simulink model "Dynamic_Model_Simulink"  (R2022a)
settings: Solver=VariableStepAuto  StartTime=0.0  StopTime=1200  MaxStep=0.001  RelTol=1e-3
values from neighbouring files (symbols this model uses):
  B_F = 10000    [Dynamic_Model.m]
  Battery_Voltage = 364    [Dynamic_Model.m]
  Cd = 0.28    [Dynamic_Model.m]
  Crr = 0.015    [Dynamic_Model.m]
  GR = 7.8    [Dynamic_Model.m]
  GVM = (Vm+Dm)    (= 1790)    [Dynamic_Model.m]
  GVW = (Vm+Dm)*g    (= 17559.9)    [Dynamic_Model.m]
  M_Eff = Motor(2:16,2:16)    [Dynamic_Model.m]
  M_Regen_Eff = Motor_Regen(2:16,2:16)    [Dynamic_Model.m]
  M_Regen_Speed = Motor_Regen(2:16,1)    [Dynamic_Model.m]
  M_Regen_Torque = Motor_Regen(2:16,17)    [Dynamic_Model.m]
  M_Speed = Motor(2:16,1)    [Dynamic_Model.m]
  M_Torque = Motor(2:16,17)    [Dynamic_Model.m]
  MC_Eff = Motor_C(2:16,2:16)    [Dynamic_Model.m]
  MC_Regen_Eff = Motor_C_Regen(2:16,2:16)    [Dynamic_Model.m]
  MC_Regen_Speed = Motor_C_Regen(2:16,1)    [Dynamic_Model.m]
  MC_Regen_Torque = Motor_C_Regen(2:16,17)    [Dynamic_Model.m]
  MC_Speed = Motor_C(2:16,1)    [Dynamic_Model.m]
  MC_Torque = Motor_C(2:16,17)    [Dynamic_Model.m]
  P_Avl = 30000    [Dynamic_Model.m]
  Rho = 1.225    [Dynamic_Model.m]
  Rw = 0.2032    [Dynamic_Model.m]
  theta = 0    [Dynamic_Model.m]
  Va = 3.8056    [Dynamic_Model.m]
libraries: slpidlib x1
settings Model: Creator=sujee  LastModifiedBy=sujee

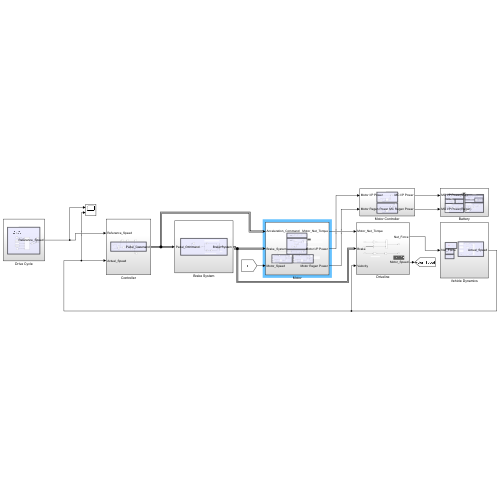
[thumbnail: Simulink's stored preview of the top-level diagram]
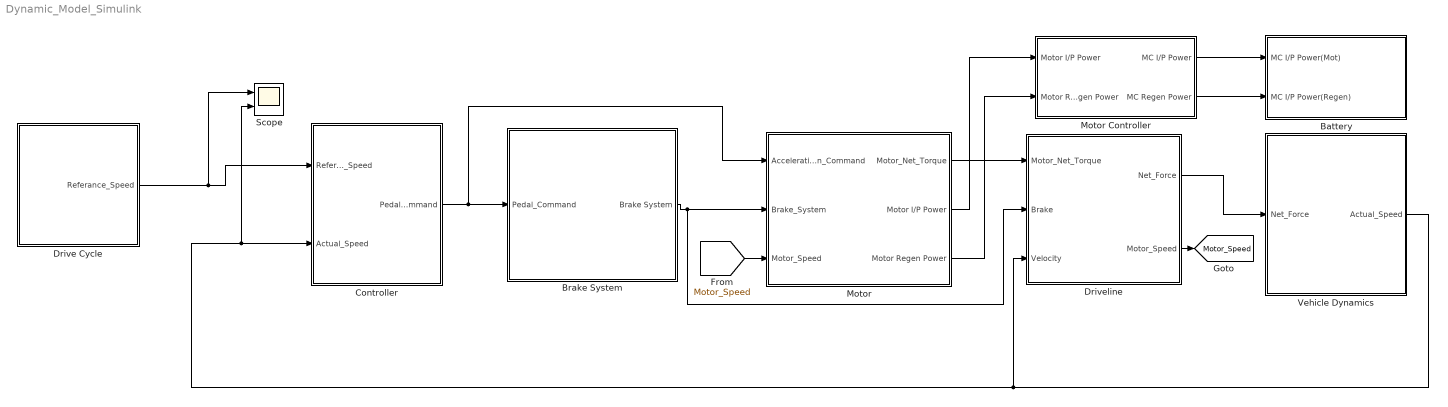
== system Dynamic_Model_Simulink ==
  Battery : Subsystem
  Brake System : Subsystem
  Controller : Subsystem
  Drive Cycle : Subsystem
  Driveline : Subsystem
  Motor : Subsystem
  Motor Controller : Subsystem
  Scope : Scope  NumInputPorts=2
  Vehicle Dynamics : Subsystem
  tag scope: Motor_Speed=global
  wires:
  Vehicle Dynamics/1(Actual_Speed) -> Scope/2, Controller/2(Actual_Speed), Driveline/3(Velocity)
  Drive Cycle/1(Referance_Speed) -> Scope/1, Controller/1(Referance_Speed)
  Controller/1(Pedal_Command) -> Motor/1(Acceleration_Command), Brake System/1(Pedal_Command)
  Brake System/1(Brake System) -> Driveline/2(Brake), Motor/2(Brake_System)
  Motor/1(Motor_Net_Torque) -> Driveline/1(Motor_Net_Torque)
  Driveline/1(Net_Force) -> Vehicle Dynamics/1(Net_Force)
  Driveline/2(Motor_Speed) -> [Motor_Speed]
  [Motor_Speed] -> Motor/3(Motor_Speed)
  Motor/2(Motor I/P Power) -> Motor Controller/1(Motor I/P Power)
  Motor/3(Motor Regen Power) -> Motor Controller/2(Motor Regen Power)
  Motor Controller/1(MC I/P Power) -> Battery/1(MC I/P Power(Mot))
  Motor Controller/2(MC Regen Power) -> Battery/2(MC I/P Power(Regen))

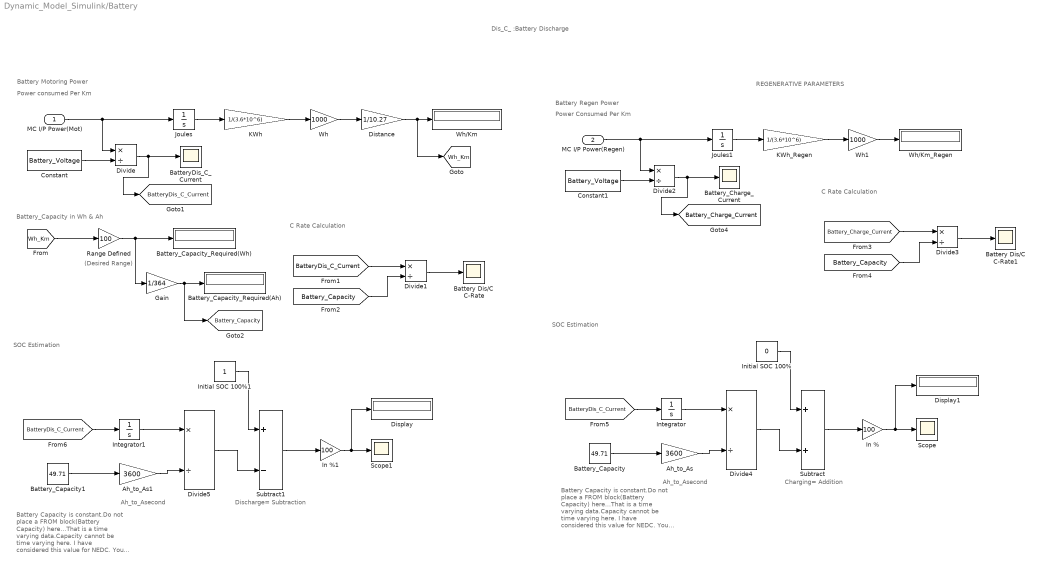
== system Dynamic_Model_Simulink/Battery ==
  note: Charging= Addition
  note: REGENERATIVE PARAMETERS
  note: SOC Estimation
  note: (Desired Range)
  note: Battery Motoring Power
  note: Battery Regen Power
  note: Dis_C_ :Battery Discharge
  note: C Rate Calculation
  note: Battery_Capacity in Wh & Ah
  note: Power consumed Per Km
  note: Power Consumed Per Km
  note: C Rate Calculation
  note: Ah_to_Asecond
  note: Battery Capacity is constant.Do not place a FROM block(Battery Capacity) here...That is a time varying data.Capacity cannot be time varying here.
      | I have considered this value for NEDC. You might get a diff value for other drive cycles, dynamically change the value here!
  note: Battery Capacity is constant.Do not place a FROM block(Battery Capacity) here...That is a time varying data.Capacity cannot be time varying here.
      | I have considered this value for NEDC. You might get a diff value for other drive cycles, dynamically change the value here!
  note: SOC Estimation
  note: Discharge= Subtraction
  note: Ah_to_Asecond
  MC I/P Power(Mot) : Inport
  MC I/P Power(Regen) : Inport  Port=2
  Ah_to_As : Gain  Gain=3600
  Ah_to_As1 : Gain  Gain=3600
  Battery Dis/C C-Rate : Scope
  Battery Dis/C C-Rate1 : Scope
  BatteryDis_C_Current : Scope
  Battery_Capacity : Constant  Value=49.71
  Battery_Capacity1 : Constant  Value=49.71
  Battery_Capacity_Required(Ah) : Display
  Battery_Capacity_Required(Wh) : Display
  Battery_Charge_Current : Scope
  Constant : Constant  Value=Battery_Voltage  VectorParams1D=off
  Constant1 : Constant  Value=Battery_Voltage  VectorParams1D=off
  Display : Display
  Display1 : Display
  Distance : Gain  Gain=1/10.27
  Divide{,1..5} (6 alike) : Product  Inputs=*/
  Gain : Gain  Gain=1/364
  In % : Gain  Gain=100
  In %1 : Gain  Gain=100
  Initial SOC 100% : Constant  Value=0
  Initial SOC 100%1 : Constant
  Integrator : Integrator
  Integrator1 : Integrator
  Joules : Integrator
  Joules1 : Integrator
  KWh : Gain  Gain=1/(3.6*10^6)
  KWh_Regen : Gain  Gain=1/(3.6*10^6)
  Range Defined : Gain  Gain=100
  Scope : Scope
  Scope1 : Scope
  Subtract : Sum
  Subtract1 : Sum  Inputs=+-
  Wh : Gain  Gain=1000
  Wh/Km : Display
  Wh/Km_Regen : Display
  Wh1 : Gain  Gain=1000
  tag scope: BatteryDis_C_Current=global, Battery_Capacity=global, Battery_Charge_Current=global, Wh_Km=global
  wires:
  MC I/P Power(Mot)/1 -> Joules/1, Divide/1
  Constant/1 -> Divide/2
  Joules/1 -> KWh/1
  KWh/1 -> Wh/1
  Wh/1 -> Distance/1
  Distance/1 -> [Wh_Km], Wh/Km/1
  [Wh_Km] -> Range Defined/1
  Range Defined/1 -> Battery_Capacity_Required(Wh)/1, Gain/1
  Divide/1 -> [BatteryDis_C_Current], BatteryDis_C_Current/1
  Gain/1 -> [Battery_Capacity], Battery_Capacity_Required(Ah)/1
  [BatteryDis_C_Current] -> Divide1/1
  [Battery_Capacity] -> Divide1/2
  Divide1/1 -> Battery Dis/C C-Rate/1
  MC I/P Power(Regen)/1 -> Joules1/1, Divide2/1
  Joules1/1 -> KWh_Regen/1
  Constant1/1 -> Divide2/2
  Divide2/1 -> [Battery_Charge_Current], Battery_Charge_Current/1
  KWh_Regen/1 -> Wh1/1
  Wh1/1 -> Wh/Km_Regen/1
  [Battery_Charge_Current] -> Divide3/1
  Divide3/1 -> Battery Dis/C C-Rate1/1
  [Battery_Capacity] -> Divide3/2
  Integrator/1 -> Divide4/1
  Battery_Capacity/1 -> Ah_to_As/1
  Initial SOC 100%/1 -> Subtract/1
  Divide4/1 -> Subtract/2
  In %/1 -> Display1/1, Scope/1
  Subtract/1 -> In %/1
  Ah_to_As/1 -> Divide4/2
  [BatteryDis_C_Current] -> Integrator/1
  Battery_Capacity1/1 -> Ah_to_As1/1
  Divide5/1 -> Subtract1/2
  Subtract1/1 -> In %1/1
  Initial SOC 100%1/1 -> Subtract1/1
  Integrator1/1 -> Divide5/1
  Ah_to_As1/1 -> Divide5/2
  [BatteryDis_C_Current] -> Integrator1/1
  In %1/1 -> Display/1, Scope1/1

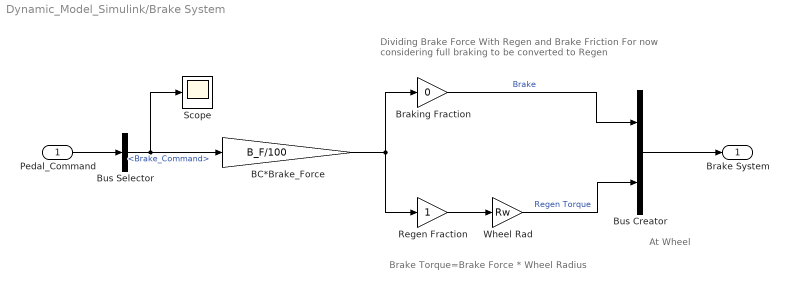
== system Dynamic_Model_Simulink/Brake System ==
  note: Dividing Brake Force With Regen and Brake Friction
      | For now considering full braking to be converted to Regen
  note: Brake Torque=Brake Force * Wheel Radius
  note: At Wheel
  Pedal_Command : Inport
  " Regen Fraction" : Gain
  BC*Brake_Force : Gain  Gain=B_F/100
  "Braking Fraction " : Gain  Gain=0
  Bus Creator : BusCreator  Inputs=2
  Bus Selector : BusSelector  OutputSignals=Brake_Command
  Scope : Scope
  Wheel Rad : Gain  Gain=Rw
  Brake System : Outport
  wires:
  Pedal_Command/1 -> Bus Selector/1
  Bus Selector/1 -> Scope/1, BC*Brake_Force/1  "<Brake_Command>"
  BC*Brake_Force/1 -> "Braking Fraction "/1, " Regen Fraction"/1
  " Regen Fraction"/1 -> Wheel Rad/1
  "Braking Fraction "/1 -> Bus Creator/1  "Brake"
  Wheel Rad/1 -> Bus Creator/2  "Regen Torque"
  Bus Creator/1 -> Brake System/1

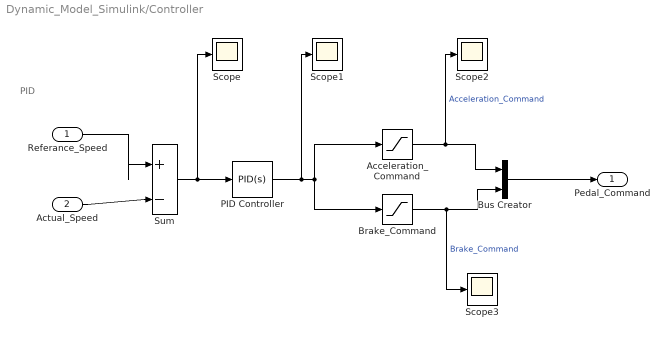
== system Dynamic_Model_Simulink/Controller ==
  note: PID
  Referance_Speed : Inport
  Actual_Speed : Inport  Port=2
  Acceleration_Command : Saturate  UpperLimit=inf  LowerLimit=0
  Brake_Command : Saturate  UpperLimit=0  LowerLimit=-inf
  Bus Creator : BusCreator  Inputs=2
  PID Controller : slpidlib/PID Controller  Controller=PID  Form=Parallel  TimeDomain=Continuous-time  UseExternalTs=off  SampleTime=-1  IntegratorMethod=Forward Euler  FilterMethod=Forward Euler  ControllerParametersSource=internal  P=200  I=1  UseKiTs=off  D=1  N=100  UseFilter=on  TunerSelectOption=Transfer Function Based (PID Tuner App)  InitialConditionSource=internal  InitialConditionForIntegrator=0  InitialConditionForFilter=0  DifferentiatorICPrevScaledInput=0  ExternalReset=none  TrackingMode=off  Kt=1  LimitOutput=off  SatLimitsSource=internal  UpperSaturationLimit=inf  LowerSaturationLimit=-inf  LinearizeAsGain=on  AntiWindupMode=none  Kb=1  POutMin=[]  POutMax=[]  IOutMin=[]  IOutMax=[]  DOutMin=[]  DOutMax=[]  NOutMin=[]  NOutMax=[]  SumOutMin=[]  SumOutMax=[]  SaturationOutMin=[]  SaturationOutMax=[]  PParamMin=[]  PParamMax=[]  IParamMin=[]  IParamMax=[]  DParamMin=[]  DParamMax=[]  NParamMin=[]  NParamMax=[]  KbParamMin=[]  KbParamMax=[]  KtParamMin=[]  KtParamMax=[]  KbOutMin=[]  KbOutMax=[]  KtOutMin=[]  KtOutMax=[]  IntegratorOutMin=[]  IntegratorOutMax=[]  FilterOutMin=[]  FilterOutMax=[]  SumI1OutMin=[]  SumI1OutMax=[]  SumI2OutMin=[]  SumI2OutMax=[]  SumI3OutMin=[]  SumI3OutMax=[]  SumI4OutMin=[]  SumI4OutMax=[]  SumDOutMin=[]  SumDOutMax=[]  DifferentiatorOutMin=[]  DifferentiatorOutMax=[]  FilterDiffOutCoefMin=[]  FilterDiffOutCoefMax=[]  ReciprocalOutMin=[]  ReciprocalOutMax=[]  SumDenOutMin=[]  SumDenOutMax=[]  SumNumOutMin=[]  SumNumOutMax=[]  DivideOutMin=[]  DivideOutMax=[]  UdiffTsProdOutMin=[]  UdiffTsProdOutMax=[]  NTsProdOutMin=[]  NTsProdOutMax=[]  UintegralTsProdOutMin=[]  UintegralTsProdOutMax=[]  UngainTsProdOutMin=[]  UngainTsProdOutMax=[]  IntegratorContinuousStateAttributes=''  IntegratorStateMustResolveToSignalObject=off  IntegratorRTWStateStorageClass=Auto  FilterContinuousStateAttributes=''  FilterStateMustResolveToSignalObject=off  FilterRTWStateStorageClass=Auto  ParallelPVariant=InternalParameters  IdealPVariant=Disabled  IVariant=InternalParameters  DVariant=InternalParameters  IntegratorVariant=Continuous  SatVariant=Disabled  AWVariant=Passthrough  PCopyVariant=Disabled  TRVariant=Disabled  FdbkBlocksVariant=Forward  IdealPFdbkVariant=Disabled  SatFdbkVariant=Disabled  DerivativeFilterVariant=ContFilter  NVariant=InternalParameters  NCopyVariant=Disabled  FilterICVariant=InternalICsFilter  IntegratorICVariant=InternalICs  ExternalResetVariant=Disabled  TRSumVariant=Passthrough  SumFdbkVariant=Disabled  SumVariant=Sum_PID  TsampFilterVariant=InternalTs  TsampNgainVariant=Passthrough  TsampIntegralVariant=Passthrough  ExternalSaturationOutDataTypeStr=Inherit: Same as second input  aMode=0
  Scope{,1..3} (4 alike) : Scope
  Sum : Sum  Inputs=|+-
  Pedal_Command : Outport
  wires:
  Referance_Speed/1 -> Sum/1
  Actual_Speed/1 -> Sum/2
  Sum/1 -> Scope/1, PID Controller/1
  PID Controller/1 -> Scope1/1, Brake_Command/1, Acceleration_Command/1
  Acceleration_Command/1 -> Scope2/1, Bus Creator/1  "Acceleration_Command"
  Brake_Command/1 -> Scope3/1, Bus Creator/2  "Brake_Command"
  Bus Creator/1 -> Pedal_Command/1

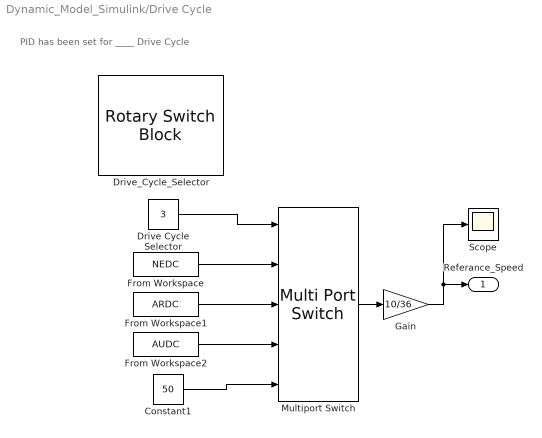
== system Dynamic_Model_Simulink/Drive Cycle ==
  note: PID has been set for ____ Drive Cycle
  Constant1 : Constant  Value=50
  Drive Cycle Selector : Constant  Value=3
  Drive_Cycle_Selector : RotarySwitchBlock
      settings: Values={{'NEDC', 'ARDC', 'AUDC', '60 m/s'}, [1 2 3 4]}
  From Workspace : FromWorkspace  VariableName=NEDC
  From Workspace1 : FromWorkspace  VariableName=ARDC
  From Workspace2 : FromWorkspace  VariableName=AUDC
  Gain : Gain  Gain=10/36
  Multiport Switch : MultiPortSwitch  Inputs=4  SaturateOnIntegerOverflow=off  InputSameDT=off
  Scope : Scope
  Referance_Speed : Outport
  wires:
  From Workspace/1 -> Multiport Switch/2
  From Workspace2/1 -> Multiport Switch/4
  From Workspace1/1 -> Multiport Switch/3
  Drive Cycle Selector/1 -> Multiport Switch/1
  Multiport Switch/1 -> Gain/1
  Constant1/1 -> Multiport Switch/5
  Gain/1 -> Scope/1, Referance_Speed/1

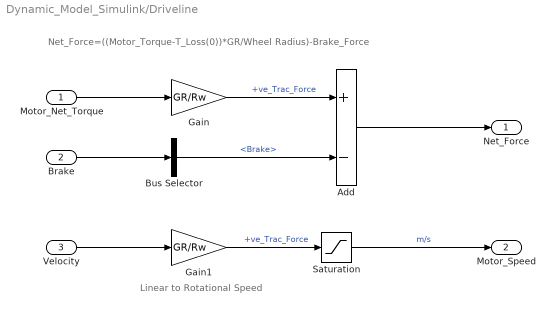
== system Dynamic_Model_Simulink/Driveline ==
  note: Linear to Rotational Speed
  note: Net_Force=((Motor_Torque-T_Loss(0))*GR/Wheel Radius)-Brake_Force
  Motor_Net_Torque : Inport
  Brake : Inport  Port=2
  Velocity : Inport  Port=3
  Add : Sum  Inputs=+-
  Bus Selector : BusSelector  OutputSignals=Brake
  Gain : Gain  Gain=GR/Rw
  Gain1 : Gain  Gain=GR/Rw
  Saturation : Saturate  UpperLimit=inf  LowerLimit=0.00001
  Net_Force : Outport
  Motor_Speed : Outport  Port=2
  wires:
  Motor_Net_Torque/1 -> Gain/1
  Gain/1 -> Add/1  "+ve_Trac_Force"
  Brake/1 -> Bus Selector/1
  Bus Selector/1 -> Add/2  "<Brake>"
  Velocity/1 -> Gain1/1
  Gain1/1 -> Saturation/1  "+ve_Trac_Force"
  Add/1 -> Net_Force/1
  Saturation/1 -> Motor_Speed/1  "m/s"

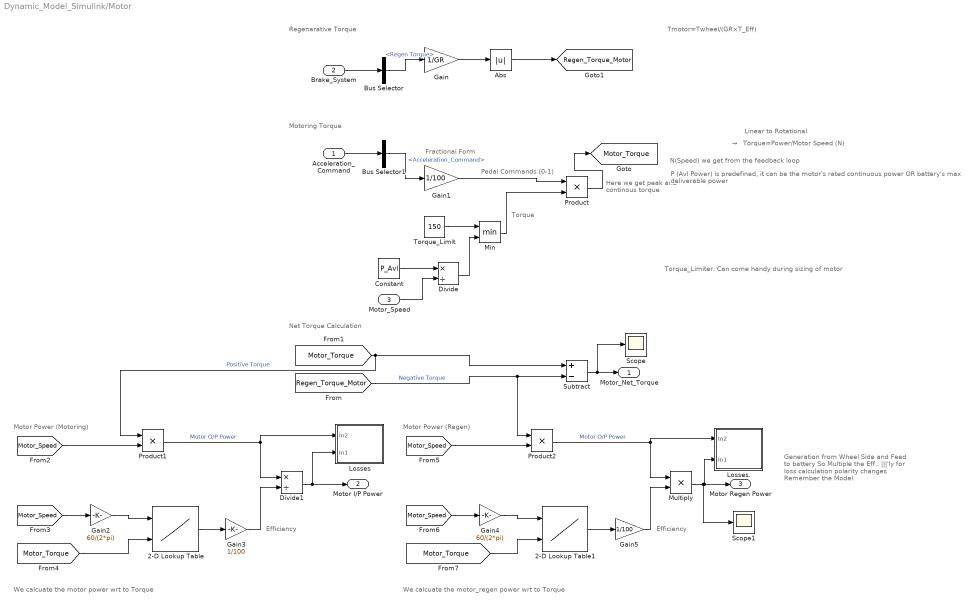
== system Dynamic_Model_Simulink/Motor ==
  note: Generation from Wheel Side and Feed to battery
      | So Multiple the Eff..
      | |||'ly for loss calculation polarity changes
      | Remember the Model.
  note: We calcuate the motor power wrt to Torque
  note: Motor Power (Motoring)
  note: Efficiency
  note: Linear to Rotational
  note: Here we get peak and continous torque
  note: Net Torque Calculation
  note: Torque
  note: P (Avl Power) is predefined, it can be the motor's rated continuous power OR battery's max deliverable power
  note: N(Speed) we get from the feedback loop
  note: →
  note: Torque=Power/Motor Speed (N)
  note: Fractional Form
  note: Motoring Torque
  note: Tmotor=Twheel​/(GR×T_Eff)
  note: Regenarative Torque
  note: Pedal Commands (0-1)
  note: Torque_Limiter: Can come handy during sizing of motor
  note: We calcuate the motor_regen power wrt to Torque
  note: Motor Power (Regen)
  note: Efficiency
  Acceleration_Command : Inport
  Brake_System : Inport  Port=2
  Motor_Speed : Inport  Port=3
  2-D Lookup Table : Lookup_n-D  BreakpointsForDimension1=M_Speed  BreakpointsForDimension2=M_Torque  Table=M_Eff  InternalRulePriority=Speed  RndMeth=Simplest
      settings: InputPortMap=u0,u1
  2-D Lookup Table1 : Lookup_n-D  BreakpointsForDimension1=M_Regen_Speed  BreakpointsForDimension2=M_Regen_Torque  Table=M_Regen_Eff  InternalRulePriority=Speed  RndMeth=Simplest
      settings: InputPortMap=u0,u1
  Abs : Abs  SaturateOnIntegerOverflow=off
  Bus Selector : BusSelector  OutputSignals=Regen Torque
  Bus Selector1 : BusSelector  OutputSignals=Acceleration_Command
  Constant : Constant  Value=P_Avl  VectorParams1D=off
  Divide : Product  Inputs=*/
  Divide1 : Product  Inputs=*/
  Gain : Gain  Gain=1/GR
  Gain1 : Gain  Gain=1/100
  Gain2 : Gain  Gain=60/(2*pi)
  Gain3 : Gain  Gain=1/100
  Gain4 : Gain  Gain=60/(2*pi)
  Gain5 : Gain  Gain=1/100
  Losses : Subsystem
  Losses. : Subsystem
  Min : MinMax  Inputs=2
  Multiply : Product  Inputs=**
  Product : Product
  Product1 : Product
  Product2 : Product
  Scope : Scope
  Scope1 : Scope
  Subtract : Sum  Inputs=+-
  Torque_Limit : Constant  Value=150  VectorParams1D=off
  Motor_Net_Torque : Outport
  Motor I/P Power : Outport  Port=2
  Motor Regen Power : Outport  Port=3
  tag scope: Motor_Torque=global, Regen_Torque_Motor=global
  wires:
  Brake_System/1 -> Bus Selector/1
  Gain/1 -> Abs/1
  Abs/1 -> [Regen_Torque_Motor]
  Bus Selector/1 -> Gain/1  "<Regen Torque>"
  Acceleration_Command/1 -> Bus Selector1/1
  Bus Selector1/1 -> Gain1/1  "<Acceleration_Command>"
  Motor_Speed/1 -> Divide/2
  Constant/1 -> Divide/1
  Divide/1 -> Min/2
  Torque_Limit/1 -> Min/1
  Min/1 -> Product/2
  Gain1/1 -> Product/1
  Product/1 -> [Motor_Torque]
  Subtract/1 -> Scope/1, Motor_Net_Torque/1
  [Motor_Torque] -> Subtract/1, Product1/1  "Positive Torque"
  [Regen_Torque_Motor] -> Product2/1, Subtract/2  "Negative Torque"
  [Motor_Speed] -> Product1/2
  [Motor_Torque] -> 2-D Lookup Table/2
  [Motor_Speed] -> Gain2/1
  Gain2/1 -> 2-D Lookup Table/1
  2-D Lookup Table/1 -> Gain3/1
  Gain3/1 -> Divide1/2
  Product1/1 -> Losses/1(In2), Divide1/1  "Motor O/P Power"
  Divide1/1 -> Losses/2(In1), Motor I/P Power/1
  Multiply/1 -> Scope1/1, Losses./2(In1), Motor Regen Power/1
  Product2/1 -> Multiply/1, Losses./1(In2)  "Motor O/P Power"
  Gain5/1 -> Multiply/2
  2-D Lookup Table1/1 -> Gain5/1
  Gain4/1 -> 2-D Lookup Table1/1
  [Motor_Speed] -> Gain4/1
  [Motor_Torque] -> 2-D Lookup Table1/2
  [Motor_Speed] -> Product2/2

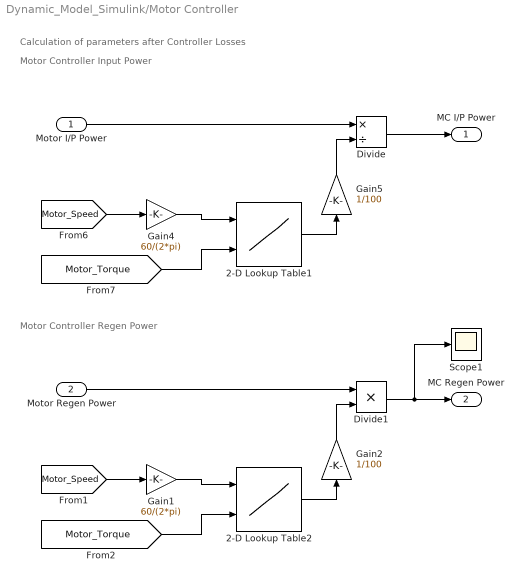
== system Dynamic_Model_Simulink/Motor Controller ==
  note: Calculation of parameters after Controller Losses
  note: Motor Controller Input Power
  note: Motor Controller Regen Power
  Motor I/P Power : Inport
  Motor Regen Power : Inport  Port=2
  2-D Lookup Table1 : Lookup_n-D  BreakpointsForDimension1=MC_Speed  BreakpointsForDimension2=MC_Torque  Table=MC_Eff  InternalRulePriority=Speed  RndMeth=Simplest
      settings: InputPortMap=u0,u1
  2-D Lookup Table2 : Lookup_n-D  BreakpointsForDimension1=MC_Regen_Speed  BreakpointsForDimension2=MC_Regen_Torque  Table=MC_Regen_Eff  InternalRulePriority=Speed  RndMeth=Simplest
      settings: InputPortMap=u0,u1
  Divide : Product  Inputs=*/
  Divide1 : Product  Inputs=**
  Gain1 : Gain  Gain=60/(2*pi)
  Gain2 : Gain  Gain=1/100
  Gain4 : Gain  Gain=60/(2*pi)
  Gain5 : Gain  Gain=1/100
  Scope1 : Scope
  MC I/P Power : Outport
  MC Regen Power : Outport  Port=2
  wires:
  Gain4/1 -> 2-D Lookup Table1/1
  [Motor_Speed] -> Gain4/1
  [Motor_Torque] -> 2-D Lookup Table1/2
  2-D Lookup Table1/1 -> Gain5/1
  Motor I/P Power/1 -> Divide/1
  Gain5/1 -> Divide/2
  Divide/1 -> MC I/P Power/1
  Gain2/1 -> Divide1/2
  Divide1/1 -> MC Regen Power/1, Scope1/1
  [Motor_Speed] -> Gain1/1
  [Motor_Torque] -> 2-D Lookup Table2/2
  Gain1/1 -> 2-D Lookup Table2/1
  2-D Lookup Table2/1 -> Gain2/1
  Motor Regen Power/1 -> Divide1/1

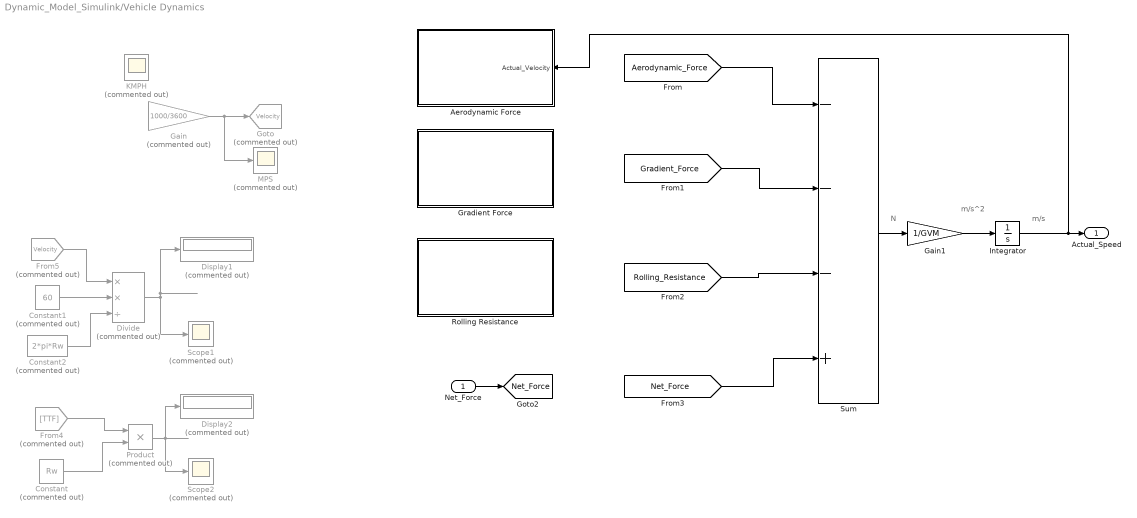
== system Dynamic_Model_Simulink/Vehicle Dynamics ==
  note: N
  note: m/s^2
  note: m/s
  Net_Force : Inport
  Aerodynamic Force : Subsystem
      settings: PortSchema="{\"entries\":[{\"content\":{\"sides\":[{\"content\":{\"connectorIds\":[]},\"type\":\"ConnectorPlacement.EquallySpacedRectSide\",\"uuid\":\"27747e7d-df0c-4666-88e2-0d7fd628eaf5\"},{\"content\":{\"connectorIds\":[\"In1\"],\"side\":\"RIGHT\"},\"type\":\"ConnectorPlacement.EquallySpacedRectSide\",\"uuid\":\"a68ab30e-bfab-45dd-a72e-c1f611b61be6\"},{\"content\":{\"connectorIds\":[],\"side\":\"TOP\"},\"type\":\"ConnectorPlacement.EquallySpacedRectSide\",\"uuid\":\"166a4daa-c768-47af-a6f7-4550d6ab2b28\"}]},\"type\":\"ConnectorPlacement.EquallySpacedConnector\",\"uuid\":\"a12af1d2-6906-497f-962e-858169b2799f\"}],\"packageUris\":[\"http://schema.mathworks.com/mf0/Connector/R2020b\"],\"version\":\"1.0\"}"
  Constant : Constant  Commented=on  Value=Rw
  Constant1 : Constant  Commented=on  Value=60
  Constant2 : Constant  Commented=on  Value=2*pi*Rw
  Display1 : Display  Commented=on
  Display2 : Display  Commented=on
  Divide : Product  Commented=on  Inputs=**/
  From4 : From  Commented=on  GotoTag=TTF  TagVisibility=global
  From5 : From  Commented=on  GotoTag=Velocity  TagVisibility=global
  Gain : Gain  Commented=on  Gain=1000/3600
  Gain1 : Gain  Gain=1/GVM
  Goto : Goto  Commented=on  GotoTag=Velocity  TagVisibility=global
  Gradient Force : Subsystem
  Integrator : Integrator
  KMPH : Scope  Commented=on
  MPS : Scope  Commented=on
  Product : Product  Commented=on
  Rolling Resistance : Subsystem
  Scope1 : Scope  Commented=on
  Scope2 : Scope  Commented=on
  Sum : Sum  Inputs=---+
  Actual_Speed : Outport
  tag scope: Net_Force=global
  wires:
  ? -> KMPH/1, Gain/1
  Gain/1 -> Goto/1, MPS/1
  [Net_Force] -> Sum/4
  [Rolling_Resistance] -> Sum/3
  [Gradient_Force] -> Sum/2
  [Aerodynamic_Force] -> Sum/1
  From4/1 -> Product/1
  Constant/1 -> Product/2
  From5/1 -> Divide/1
  Constant1/1 -> Divide/2
  Constant2/1 -> Divide/3
  Divide/1 -> Display1/1, Scope1/1
  Product/1 -> Scope2/1, Display2/1
  Net_Force/1 -> [Net_Force]
  Sum/1 -> Gain1/1
  Gain1/1 -> Integrator/1
  Integrator/1 -> Aerodynamic Force/1(Actual_Velocity), Actual_Speed/1

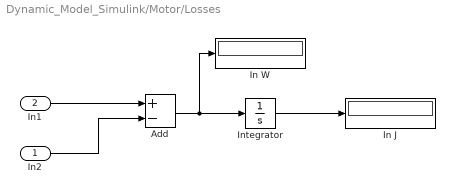
== system Dynamic_Model_Simulink/Motor/Losses ==
  In2 : Inport
  In1 : Inport  Port=2
  Add : Sum  Inputs=+-
  In J : Display
  In W : Display
  Integrator : Integrator
  wires:
  In1/1 -> Add/1
  In2/1 -> Add/2
  Add/1 -> In W/1, Integrator/1
  Integrator/1 -> In J/1

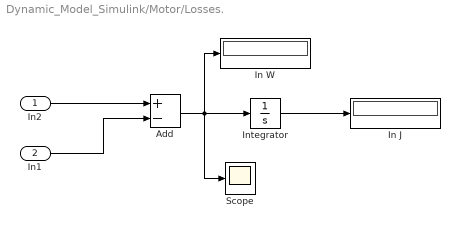
== system Dynamic_Model_Simulink/Motor/Losses. ==
  In2 : Inport
  In1 : Inport  Port=2
  Add : Sum  Inputs=+-
  In J : Display
  In W : Display
  Integrator : Integrator
  Scope : Scope
  wires:
  In2/1 -> Add/1
  In1/1 -> Add/2
  Add/1 -> Scope/1, In W/1, Integrator/1
  Integrator/1 -> In J/1

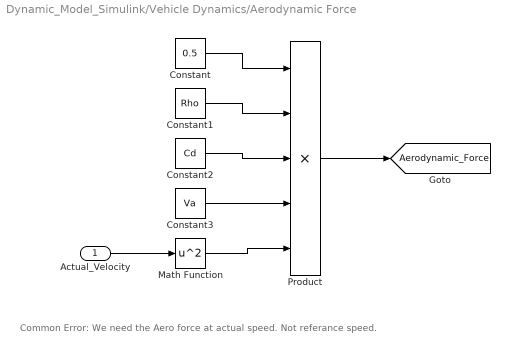
== system Dynamic_Model_Simulink/Vehicle Dynamics/Aerodynamic Force ==
  note: Common Error: We need the Aero force at actual speed. Not referance speed.
  Actual_Velocity : Inport
  Constant : Constant  Value=0.5
  Constant1 : Constant  Value=Rho
  Constant2 : Constant  Value=Cd
  Constant3 : Constant  Value=Va
  Math Function : Math  Operator=square
  Product : Product  Inputs=5
  tag scope: Aerodynamic_Force=global
  wires:
  Actual_Velocity/1 -> Math Function/1
  Constant/1 -> Product/1
  Constant1/1 -> Product/2
  Constant2/1 -> Product/3
  Constant3/1 -> Product/4
  Math Function/1 -> Product/5
  Product/1 -> [Aerodynamic_Force]

== system Dynamic_Model_Simulink/Vehicle Dynamics/Gradient Force ==
  Constant : Constant  Value=GVW
  Constant1 : Constant  Value=theta
  Display : Display
  Product : Product
  Scope : Scope
  tag scope: Gradient_Force=global
  wires:
  Constant/1 -> Product/1
  Constant1/1 -> Product/2
  Product/1 -> Scope/1, Display/1, [Gradient_Force]

== system Dynamic_Model_Simulink/Vehicle Dynamics/Rolling Resistance ==
  Constant : Constant  Value=GVW
  Constant1 : Constant  Value=Crr
  Display : Display
  Product : Product
  Scope : Scope
  tag scope: Rolling_Resistance=global
  wires:
  Constant/1 -> Product/1
  Constant1/1 -> Product/2
  Product/1 -> Display/1, Scope/1, [Rolling_Resistance]
